simulink model "pTopModel"  (R2021a)
settings: Solver=FixedStepAuto  StartTime=0.0  StopTime=200  FixedStep=Ts  RelTol=1e-3
values from neighbouring files (symbols this model uses):
  C = 1 - 0.287*log(gamma)    [SIDWaveGenerator.m]
  Ef = rho*g^2*D*A^2/(4*w)    [SIDWaveGenerator.m]
  Ts = 1/1000    (= 0.001)    [FOSTWINctrlPost.m]    (also in initModels_GUI.m)
undefined symbols (not defined in the file or in its folder): Aft, AveragePower, Bow, dataID_twin, pcktID, SimStateMsg, Total
libraries: simulink x19, slrealtimeutilitieslib x11, slrealtimeethercatlib x6, slrealtimeiplib x3, slrealtimeloglib x2, dspstat3 x1
settings Model: SimulationMode=external  Creator=Johannes  LastModifiedBy=HWRL user
settings SolverCC: ConcurrentTasks=on  AlgebraicLoopSolver=TrustRegion  PositivePriorityOrder=on
settings DataIOCC: ExternalInput=Fexin.getElement(1),Fexin.getElement(2)  LoadExternalInput=on
settings OptimizationCC: BlockReduction=off  OptimizeBlockIOStorage=off
settings DebuggingCC: TasksWithSamePriorityMsg=none  SFMachineParentedDataDiag=warning
settings HardwareCC: ProdBitPerLong=64  ProdLongLongMode=on  ProdHWDeviceType=Intel->x86-64 (Linux 64)
settings RTWCC: Description=Simulink Real-Time  SystemTargetFile=slrealtime.tlc  TemplateMakefile=slrealtime_default_tmf  RTWVerbose=off  Toolchain=Simulink Real-Time Toolchain  BuildConfiguration=Faster Runs  CodeExecutionProfiling=on  TargetLang=C++

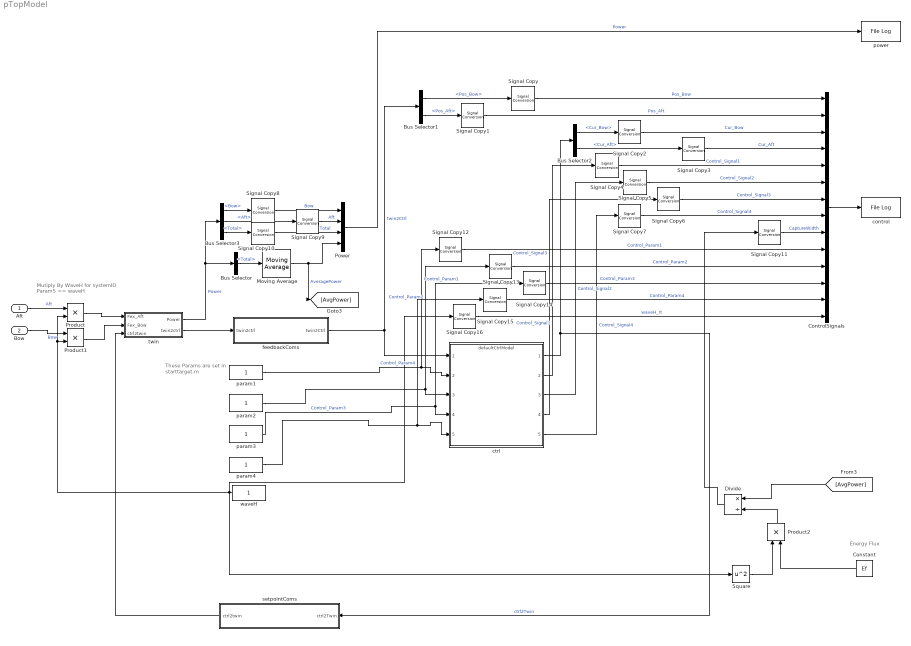
== system pTopModel ==
  note: Energy Flux
  note: Mutiply By WaveH for systemID
      | Param5 == waveH
  note: These Params are set in starttarget.m
  Aft : Inport  Interpolate=off
  Bow : Inport  Port=2  Interpolate=off
  Bus Selector : BusSelector  OutputSignals=Total
  Bus Selector1 : BusSelector  OutputSignals=Pos_Bow,Pos_Aft
  Bus Selector2 : BusSelector  OutputSignals=Cur_Bow,Cur_Aft
  Bus Selector3 : BusSelector  OutputSignals=Bow,Aft,Total
  Constant : Constant  Value=Ef  SampleTime=Ts
  ControlSignals : BusCreator  Inputs=14
  Divide : Product  Inputs=*/
  Moving Average : dspstat3/Moving Average  Method=Sliding window  ForgettingFactorPort=off  SpecifyWindowLength=on  WindowLength=numSteps  ForgettingFactor=0.9  SimulateUsing=Code generation
  Power : BusCreator  Inputs=Bow,Aft,Total,AveragePower
  Product : Product
  Product1 : Product
  Product2 : Product
  Signal Copy{,1..16} (17 alike) : SignalConversion  OverrideOpt=off
  Square : Math  Operator=square  SaturateOnIntegerOverflow=on
  control : slrealtimeloglib/File Log  decimation=10
      settings: SourceProductBaseCode=XP
  ctrl : ModelReference  ModelNameDialog=defaultCtrlModel  SimulationMode=Normal  ModelReferenceVersion=2.693
  feedbackComs : Subsystem  Variant=on  VariantControlMode=label  LabelModeActiveChoice=singleSpeedgoat
  param1 : Constant  OutDataTypeStr=Inherit: Inherit via back propagation  SampleTime=Ts
  param2 : Constant  SampleTime=Ts
  param3 : Constant  SampleTime=Ts
  param4 : Constant  VectorParams1D=off  SampleTime=Ts
  power : slrealtimeloglib/File Log  decimation=10
      settings: SourceProductBaseCode=XP
  setpointComs : Subsystem  Variant=on  VariantControlMode=label  LabelModeActiveChoice=singleSpeedgoat
  twin : Subsystem  Variant=on  VariantControlMode=label  LabelModeActiveChoice=systemID
  waveH : Constant  SampleTime=Ts
  wires:
  ctrl/1 -> Bus Selector2/1, setpointComs/1(ctrl2Twin)  "ctrl2Twin"
  feedbackComs/1(twin2Ctrl) -> ctrl/1, Bus Selector1/1  "twin2Ctrl"
  param1/1 -> ctrl/2, Signal Copy12/1  "Control_Param1"
  param2/1 -> ctrl/3, Signal Copy13/1  "Control_Param2"
  setpointComs/1(ctrl2twin) -> twin/3(ctrl2twin)
  twin/2(twin2ctrl) -> feedbackComs/1(twin2ctrl)
  param3/1 -> ctrl/4, Signal Copy14/1  "Control_Param3"
  ctrl/2 -> Signal Copy4/1  "Control_Signal1"
  ctrl/3 -> Signal Copy5/1  "Control_Signal2"
  ctrl/4 -> Signal Copy6/1  "Control_Signal3"
  ControlSignals/1 -> control/1
  param4/1 -> ctrl/5, Signal Copy15/1  "Control_Param4"
  Aft/1 -> Product/1  "Aft"
  Product/1 -> twin/1(Fex_Aft)
  Bow/1 -> Product1/1  "Bow"
  Product1/1 -> twin/2(Fex_Bow)
  ctrl/5 -> Signal Copy7/1  "Control_Signal4"
  twin/1(Power) -> Bus Selector3/1, Bus Selector/1  "Power"
  Bus Selector/1 -> Moving Average/1  "<Total>"
  Moving Average/1 -> [AvgPower], Power/4  "AveragePower"
  Power/1 -> power/1  "Power"
  Bus Selector1/1 -> Signal Copy/1  "<Pos_Bow>"
  Bus Selector1/2 -> Signal Copy1/1  "<Pos_Aft>"
  Bus Selector2/1 -> Signal Copy2/1  "<Cur_Bow>"
  Bus Selector2/2 -> Signal Copy3/1  "<Cur_Aft>"
  Bus Selector3/3 -> Signal Copy10/1  "<Total>"
  Bus Selector3/2 -> Signal Copy9/1  "<Aft>"
  Bus Selector3/1 -> Signal Copy8/1  "<Bow>"
  Signal Copy/1 -> ControlSignals/1  "Pos_Bow"
  Signal Copy1/1 -> ControlSignals/2  "Pos_Aft"
  Signal Copy2/1 -> ControlSignals/3  "Cur_Bow"
  Signal Copy3/1 -> ControlSignals/4  "Cur_Aft"
  Signal Copy4/1 -> ControlSignals/5  "Control_Signal1"
  Signal Copy5/1 -> ControlSignals/6  "Control_Signal2"
  Signal Copy6/1 -> ControlSignals/7  "Control_Signal3"
  Signal Copy7/1 -> ControlSignals/8  "Control_Signal4"
  Signal Copy8/1 -> Power/1  "Bow"
  Signal Copy9/1 -> Power/2  "Aft"
  Signal Copy10/1 -> Power/3  "Total"
  [AvgPower] -> Divide/1
  Constant/1 -> Product2/2
  Square/1 -> Product2/1
  Product2/1 -> Divide/2
  Divide/1 -> Signal Copy11/1
  Signal Copy11/1 -> ControlSignals/9  "CaptureWidth"
  Signal Copy12/1 -> ControlSignals/10  "Control_Param1"
  Signal Copy13/1 -> ControlSignals/11  "Control_Param2"
  Signal Copy14/1 -> ControlSignals/12  "Control_Param3"
  Signal Copy15/1 -> ControlSignals/13  "Control_Param4"
  Signal Copy16/1 -> ControlSignals/14  "waveH_rt"
  waveH/1 -> Square/1, Product/2, Product1/2, Signal Copy16/1

== system pTopModel/feedbackComs ==
  note: 1) Add Subsystem or Model blocks as valid variant choices.
      | 2) You cannot connect blocks at this level. At simulation, connectivity is automatically
      | determined, based on the active variant and port name matching.
  twin2ctrl : Inport
  nonRT : Subsystem  VariantControl=nonRT
  singleSpeedgoat : Subsystem  VariantControl=singleSpeedgoat
  twoSpeedgoats : Subsystem  VariantControl=twoSpeedgoats
  twin2Ctrl : Outport

== system pTopModel/setpointComs ==
  note: 1) Add Subsystem or Model blocks as valid variant choices.
      | 2) You cannot connect blocks at this level. At simulation, connectivity is automatically
      | determined, based on the active variant and port name matching.
  ctrl2Twin : Inport
  nonRT : Subsystem  VariantControl=nonRT
  singleSpeedgoat : Subsystem  VariantControl=singleSpeedgoat
  twoSpeedgoats : Subsystem  VariantControl=twoSpeedgoats
  ctrl2twin : Outport

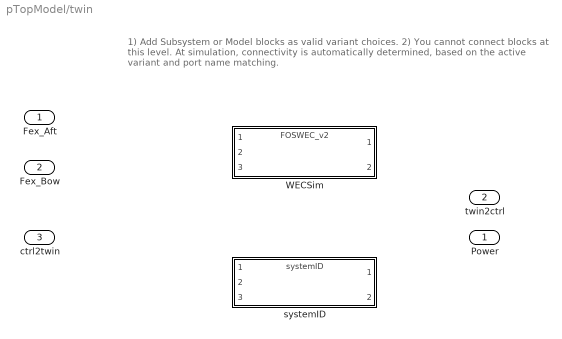
== system pTopModel/twin ==
  note: 1) Add Subsystem or Model blocks as valid variant choices.
      | 2) You cannot connect blocks at this level. At simulation, connectivity is automatically
      | determined, based on the active variant and port name matching.
  Fex_Aft : Inport
  Fex_Bow : Inport  Port=2
  ctrl2twin : Inport  Port=3
  WECSim : ModelReference  ModelNameDialog=FOSWEC_v2.slx  SimulationMode=Normal  VariantControl=WECSim  ModelReferenceVersion=3.577
  systemID : ModelReference  ModelNameDialog=systemID.slx  SimulationMode=Normal  VariantControl=systemID  ModelReferenceVersion=1.369
  Power : Outport
  twin2ctrl : Outport  Port=2

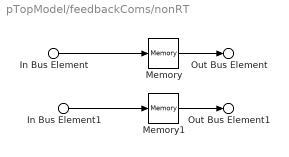
== system pTopModel/feedbackComs/nonRT ==
  In Bus Element : Inport  PortName=twin2ctrl  Element=Pos_Bow
  In Bus Element1 : Inport  PortName=twin2ctrl  Element=Pos_Aft
  Memory : Memory
  Memory1 : Memory
  Out Bus Element : Outport  PortName=twin2Ctrl  Element=Pos_Bow
  Out Bus Element1 : Outport  PortName=twin2Ctrl  Element=Pos_Aft
  wires:
  In Bus Element/1 -> Memory/1
  In Bus Element1/1 -> Memory1/1
  Memory1/1 -> Out Bus Element1/1
  Memory/1 -> Out Bus Element/1

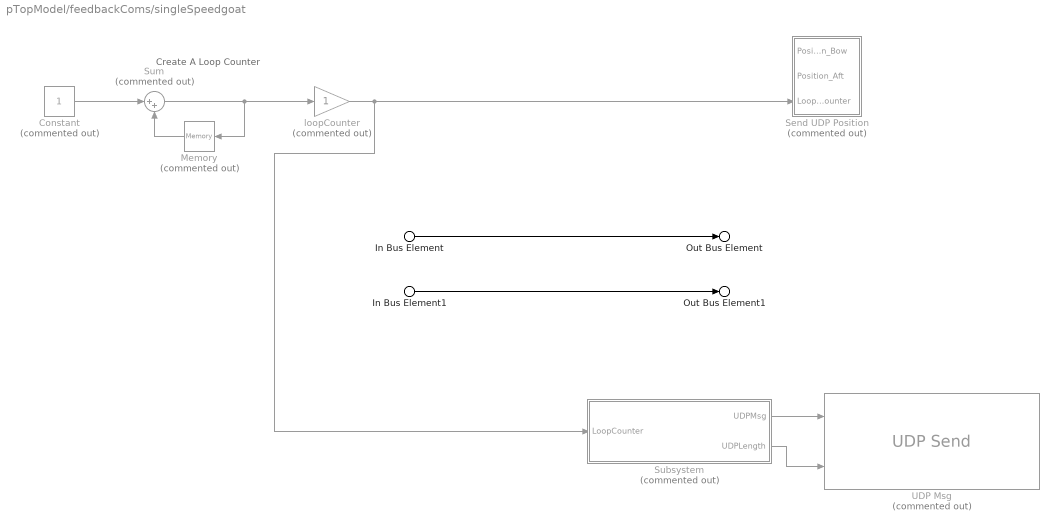
== system pTopModel/feedbackComs/singleSpeedgoat ==
  note: Create A Loop Counter
  In Bus Element : Inport  PortName=twin2ctrl  Element=Pos_Bow
  In Bus Element1 : Inport  PortName=twin2ctrl  Element=Pos_Aft
  Constant : Constant  Commented=on  SampleTime=Ts
  Memory : Memory  Commented=on
  Send UDP Position : Subsystem  Commented=on
  Subsystem : Subsystem  Commented=on
  Sum : Sum  Commented=on  Inputs=|++  OutDataTypeStr=uint32
  UDP Msg : slrealtimeiplib/UDP Send  Commented=on  useHostTargetConn=on  ipAddress=10.10.10.15  localPort=iotLocalMsgPort  toAddress=iotIPaddr  toPort=iotRemoteMsgPort  sampleTime=Ts
      settings: SourceProductBaseCode=XP
  loopCounter : Gain  Commented=on  ParamDataTypeStr=uint32  OutDataTypeStr=uint32
  Out Bus Element : Outport  PortName=twin2Ctrl  Element=Pos_Bow
  Out Bus Element1 : Outport  PortName=twin2Ctrl  Element=Pos_Aft
  wires:
  Subsystem/1(UDPMsg) -> UDP Msg/1
  Subsystem/2(UDPLength) -> UDP Msg/2
  In Bus Element/1 -> Out Bus Element/1
  In Bus Element1/1 -> Out Bus Element1/1
  Constant/1 -> Sum/1
  Sum/1 -> Memory/1, loopCounter/1
  Memory/1 -> Sum/2
  loopCounter/1 -> Subsystem/1(LoopCounter), Send UDP Position/3(LoopCounter)

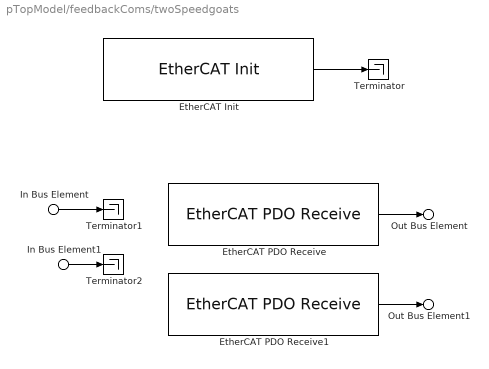
== system pTopModel/feedbackComs/twoSpeedgoats ==
  In Bus Element : Inport  PortName=twin2ctrl  Element=Pos_Bow
  In Bus Element1 : Inport  PortName=twin2ctrl  Element=Pos_Aft
  EtherCAT Init : slrealtimeethercatlib/EtherCAT Init  Priority=0  config_file=C:\Software\FOSTWIN\esi\FOSTWIN_Secondary1.xml  device_id=0  pci_bus=0  pci_slot=0  pci_function=0  portnum=1  initstate=2  dctuning=2  enaDebug=2  enaDC=on  errLink=off  masterDbg=off  stateChgDbg=off  baseClock=off  masterCfg=off  logFile='c:\dbglog.txt'  sample_time=0.001000  DCMode=0
      settings: SourceProductBaseCode=XP
  EtherCAT PDO Receive : slrealtimeethercatlib/EtherCAT PDO Receive  Priority=2  sig_name=Box 1 (EL6695-0002).IO Inputs.P2S01  sig_offset=328  sig_type=double  type_size=64  sig_dim=1  device_id=0  sample_time=0.001000
      settings: SourceProductBaseCode=XP
  EtherCAT PDO Receive1 : slrealtimeethercatlib/EtherCAT PDO Receive  Priority=2  sig_name=Box 1 (EL6695-0002).IO Inputs.P2S02  sig_offset=392  sig_type=double  type_size=64  sig_dim=1  device_id=0  sample_time=0.001000
      settings: SourceProductBaseCode=XP
  Terminator : Terminator
  Terminator1 : Terminator
  Terminator2 : Terminator
  Out Bus Element : Outport  PortName=twin2Ctrl  Element=Pos_Bow
  Out Bus Element1 : Outport  PortName=twin2Ctrl  Element=Pos_Aft
  wires:
  EtherCAT Init/1 -> Terminator/1
  EtherCAT PDO Receive/1 -> Out Bus Element/1
  In Bus Element/1 -> Terminator1/1
  EtherCAT PDO Receive1/1 -> Out Bus Element1/1
  In Bus Element1/1 -> Terminator2/1

== system pTopModel/setpointComs/nonRT ==
  In Bus Element : Inport  PortName=ctrl2Twin  Element=Cur_Bow
  In Bus Element1 : Inport  PortName=ctrl2Twin  Element=Cur_Aft
  Out Bus Element : Outport  PortName=ctrl2twin  Element=Cur_Bow
  Out Bus Element1 : Outport  PortName=ctrl2twin  Element=Cur_Aft
  wires:
  In Bus Element/1 -> Out Bus Element/1
  In Bus Element1/1 -> Out Bus Element1/1

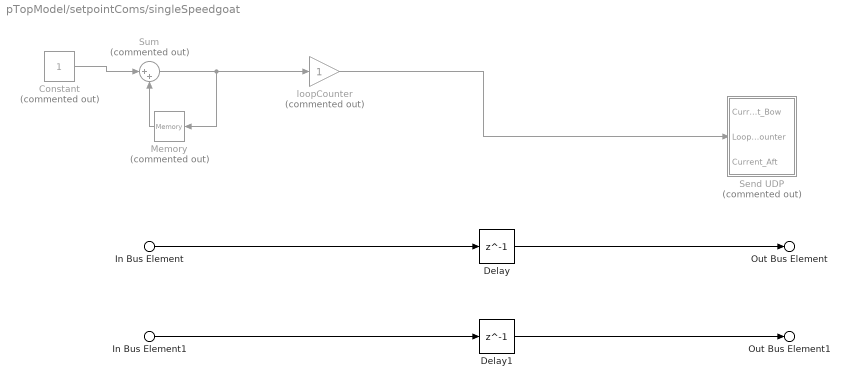
== system pTopModel/setpointComs/singleSpeedgoat ==
  In Bus Element : Inport  PortName=ctrl2Twin  Element=Cur_Bow
  In Bus Element1 : Inport  PortName=ctrl2Twin  Element=Cur_Aft
  Constant : Constant  Commented=on  SampleTime=Ts
  Delay : Delay  DelayLength=1
  Delay1 : Delay  DelayLength=1
  Memory : Memory  Commented=on
  Send UDP : Subsystem  Commented=on
  Sum : Sum  Commented=on  Inputs=|++  OutDataTypeStr=uint32
  loopCounter : Gain  Commented=on  ParamDataTypeStr=uint32  OutDataTypeStr=uint32
  Out Bus Element : Outport  PortName=ctrl2twin  Element=Cur_Bow
  Out Bus Element1 : Outport  PortName=ctrl2twin  Element=Cur_Aft
  wires:
  Constant/1 -> Sum/1
  In Bus Element/1 -> Delay/1
  In Bus Element1/1 -> Delay1/1
  Delay/1 -> Out Bus Element/1
  Delay1/1 -> Out Bus Element1/1
  Sum/1 -> Memory/1, loopCounter/1
  Memory/1 -> Sum/2
  loopCounter/1 -> Send UDP/2(LoopCounter)

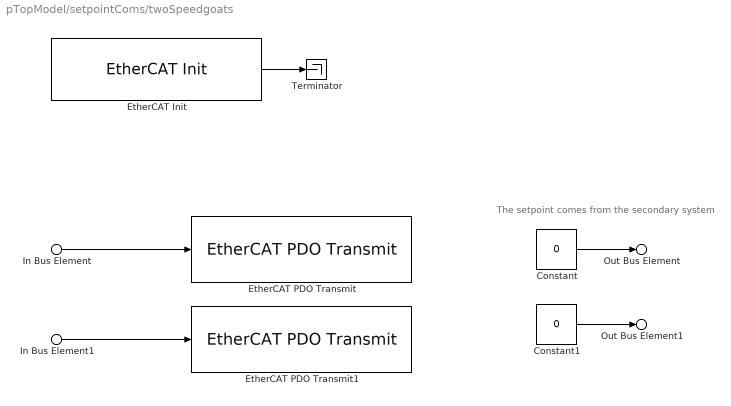
== system pTopModel/setpointComs/twoSpeedgoats ==
  note: The setpoint comes from the secondary system
  In Bus Element : Inport  PortName=ctrl2Twin  Element=Cur_Bow
  In Bus Element1 : Inport  PortName=ctrl2Twin  Element=Cur_Aft
  Constant : Constant  Value=0  VectorParams1D=off  SampleTime=-1
  Constant1 : Constant  Value=0  VectorParams1D=off  SampleTime=-1
  EtherCAT Init : slrealtimeethercatlib/EtherCAT Init  Priority=0  config_file=C:\Software\FOSTWIN\esi\FOSTWIN-Primary1.xml  device_id=0  pci_bus=0  pci_slot=0  pci_function=0  portnum=1  initstate=2  dctuning=0  enaDebug=0  enaDC=on  errLink=off  masterDbg=off  stateChgDbg=off  baseClock=off  masterCfg=off  logFile='c:\dbglog.txt'  sample_time=0.001000  DCMode=0
      settings: SourceProductBaseCode=XP
  EtherCAT PDO Transmit : slrealtimeethercatlib/EtherCAT PDO Transmit  Priority=3  sig_name=Term 2 (EL6695).IO Outputs.P2S01  sig_offset=312  sig_type=double  type_size=64  sig_dim=1  device_id=0  sample_time=0.001000
      settings: SourceProductBaseCode=XP
  EtherCAT PDO Transmit1 : slrealtimeethercatlib/EtherCAT PDO Transmit  Priority=3  sig_name=Term 2 (EL6695).IO Outputs.P2S02  sig_offset=376  sig_type=double  type_size=64  sig_dim=1  device_id=0  sample_time=0.001000
      settings: SourceProductBaseCode=XP
  Terminator : Terminator
  Out Bus Element : Outport  PortName=ctrl2twin  Element=Cur_Bow
  Out Bus Element1 : Outport  PortName=ctrl2twin  Element=Cur_Aft
  wires:
  Constant/1 -> Out Bus Element/1
  EtherCAT Init/1 -> Terminator/1
  Constant1/1 -> Out Bus Element1/1
  In Bus Element1/1 -> EtherCAT PDO Transmit1/1
  In Bus Element/1 -> EtherCAT PDO Transmit/1

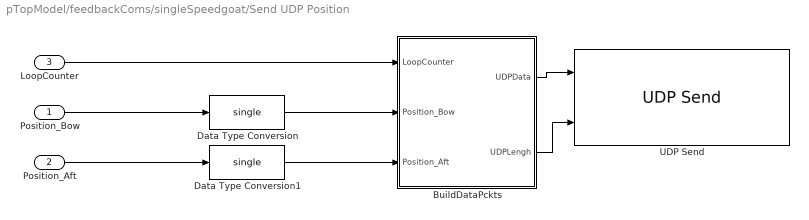
== system pTopModel/feedbackComs/singleSpeedgoat/Send UDP Position ==
  Position_Bow : Inport
  Position_Aft : Inport  Port=2
  LoopCounter : Inport  Port=3
  BuildDataPckts : Subsystem
  Data Type Conversion : DataTypeConversion  OutDataTypeStr=single
  Data Type Conversion1 : DataTypeConversion  OutDataTypeStr=single
  UDP Send : slrealtimeiplib/UDP Send  useHostTargetConn=on  ipAddress=10.10.10.15  localPort=iotLocalDataPort  toAddress=iotIPaddr  toPort=iotRemoteDataPort  sampleTime=Ts
      settings: SourceProductBaseCode=XP
  wires:
  BuildDataPckts/1(UDPData) -> UDP Send/1
  BuildDataPckts/2(UDPLengh) -> UDP Send/2
  Position_Bow/1 -> Data Type Conversion/1
  Data Type Conversion/1 -> BuildDataPckts/2(Position_Bow)
  Position_Aft/1 -> Data Type Conversion1/1
  Data Type Conversion1/1 -> BuildDataPckts/3(Position_Aft)
  LoopCounter/1 -> BuildDataPckts/1(LoopCounter)

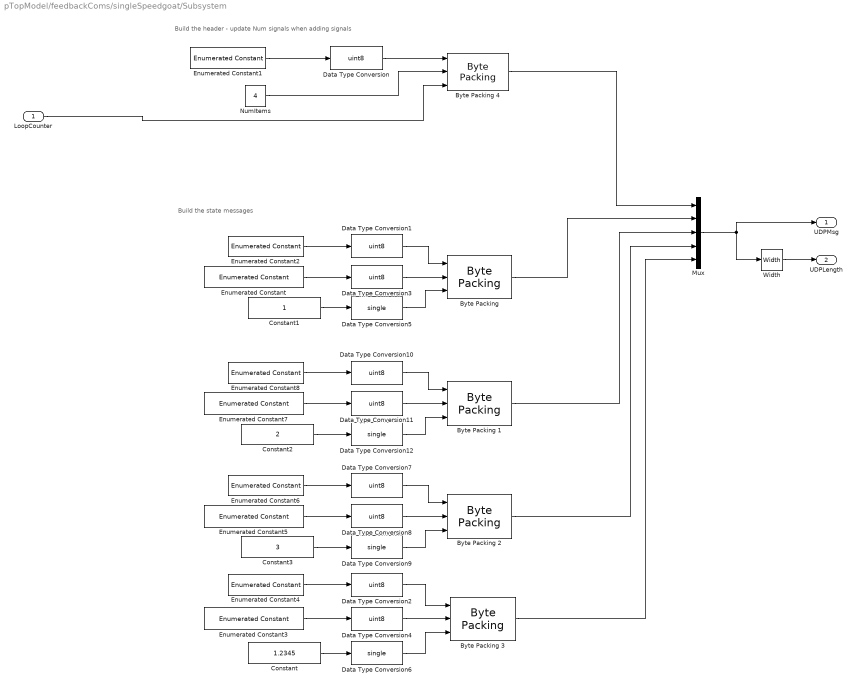
== system pTopModel/feedbackComs/singleSpeedgoat/Subsystem ==
  note: Build the state messages
  note: Build the header - update Num signals when adding signals
  LoopCounter : Inport
  Byte Packing {,1..4} (5 alike) : slrealtimeutilitieslib/Byte Packing
  Constant : Constant  Value=1.2345
  Constant1 : Constant
  Constant2 : Constant  Value=2
  Constant3 : Constant  Value=3
  Data Type Conversion{,1..4,7..8,10..11} (9 alike) : DataTypeConversion  OutDataTypeStr=uint8
  Data Type Conversion{5..6,9,12} (4 alike) : DataTypeConversion  OutDataTypeStr=single
  Enumerated Constant : simulink/Sources/Enumerated Constant  OutDataTypeStr=Enum: SimStateMsg  Value=SimStateMsg.eCATState  SampleTime=inf
  Enumerated Constant1 : simulink/Sources/Enumerated Constant  OutDataTypeStr=Enum: pcktID  Value=pcktID.header  SampleTime=inf
  Enumerated Constant{2,4,6,8} (4 alike) : simulink/Sources/Enumerated Constant  OutDataTypeStr=Enum: pcktID  Value=pcktID.stateMsg  SampleTime=inf
  Enumerated Constant3 : simulink/Sources/Enumerated Constant  OutDataTypeStr=Enum: SimStateMsg  Value=SimStateMsg.cpuTET  SampleTime=inf
  Enumerated Constant5 : simulink/Sources/Enumerated Constant  OutDataTypeStr=Enum: SimStateMsg  Value=SimStateMsg.eCATLastErr  SampleTime=inf
  Enumerated Constant7 : simulink/Sources/Enumerated Constant  OutDataTypeStr=Enum: SimStateMsg  Value=SimStateMsg.eCATErr  SampleTime=inf
  Mux : Mux  Inputs=5
  NumItems : Constant  Value=4  OutDataTypeStr=uint8
  Width : Width
  UDPMsg : Outport
  UDPLength : Outport  Port=2
  wires:
  Constant2/1 -> Data Type Conversion12/1
  NumItems/1 -> Byte Packing 4/2
  Data Type Conversion9/1 -> Byte Packing 2/3
  Constant3/1 -> Data Type Conversion9/1
  Enumerated Constant2/1 -> Data Type Conversion1/1
  Constant1/1 -> Data Type Conversion5/1
  Enumerated Constant7/1 -> Data Type Conversion11/1
  Data Type Conversion2/1 -> Byte Packing 3/1
  Enumerated Constant4/1 -> Data Type Conversion2/1
  Data Type Conversion4/1 -> Byte Packing 3/2
  Enumerated Constant6/1 -> Data Type Conversion7/1
  Mux/1 -> UDPMsg/1, Width/1
  Byte Packing 1/1 -> Mux/3
  Width/1 -> UDPLength/1
  Data Type Conversion5/1 -> "Byte Packing "/3
  Data Type Conversion12/1 -> Byte Packing 1/3
  "Byte Packing "/1 -> Mux/2
  Data Type Conversion3/1 -> "Byte Packing "/2
  Data Type Conversion6/1 -> Byte Packing 3/3
  Data Type Conversion8/1 -> Byte Packing 2/2
  Enumerated Constant3/1 -> Data Type Conversion4/1
  Enumerated Constant8/1 -> Data Type Conversion10/1
  Data Type Conversion11/1 -> Byte Packing 1/2
  Enumerated Constant5/1 -> Data Type Conversion8/1
  Data Type Conversion1/1 -> "Byte Packing "/1
  Byte Packing 4/1 -> Mux/1
  Byte Packing 3/1 -> Mux/5
  Byte Packing 2/1 -> Mux/4
  Enumerated Constant/1 -> Data Type Conversion3/1
  Constant/1 -> Data Type Conversion6/1
  Data Type Conversion10/1 -> Byte Packing 1/1
  Data Type Conversion/1 -> Byte Packing 4/1
  Data Type Conversion7/1 -> Byte Packing 2/1
  Enumerated Constant1/1 -> Data Type Conversion/1
  LoopCounter/1 -> Byte Packing 4/3

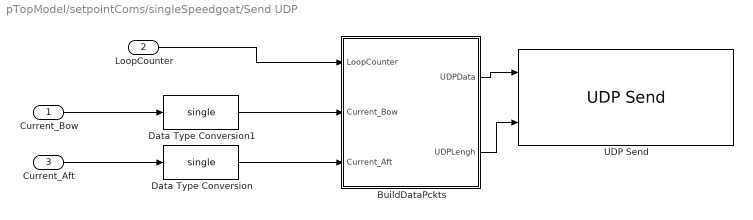
== system pTopModel/setpointComs/singleSpeedgoat/Send UDP ==
  Current_Bow : Inport
  LoopCounter : Inport  Port=2
  Current_Aft : Inport  Port=3
  BuildDataPckts : Subsystem
  Data Type Conversion : DataTypeConversion  OutDataTypeStr=single
  Data Type Conversion1 : DataTypeConversion  OutDataTypeStr=single
  UDP Send : slrealtimeiplib/UDP Send  useHostTargetConn=on  ipAddress=10.10.10.15  localPort=iotLocalDataPort  toAddress=iotIPaddr  toPort=iotRemoteDataPort  sampleTime=Ts
      settings: SourceProductBaseCode=XP
  wires:
  Current_Bow/1 -> Data Type Conversion1/1
  BuildDataPckts/1(UDPData) -> UDP Send/1
  BuildDataPckts/2(UDPLengh) -> UDP Send/2
  Current_Aft/1 -> Data Type Conversion/1
  LoopCounter/1 -> BuildDataPckts/1(LoopCounter)
  Data Type Conversion1/1 -> BuildDataPckts/2(Current_Bow)
  Data Type Conversion/1 -> BuildDataPckts/3(Current_Aft)

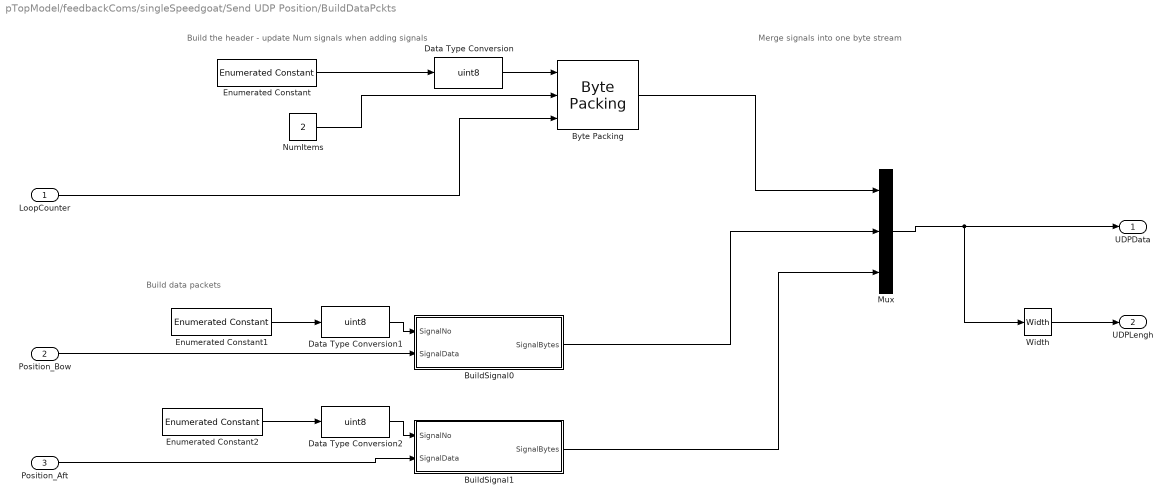
== system pTopModel/feedbackComs/singleSpeedgoat/Send UDP Position/BuildDataPckts ==
  note: Merge signals into one byte stream
  note: Build data packets
  note: Build the header - update Num signals when adding signals
  LoopCounter : Inport
  Position_Bow : Inport  Port=2  OutDataTypeStr=single
  Position_Aft : Inport  Port=3  OutDataTypeStr=single
  BuildSignal0 : Subsystem
  BuildSignal1 : Subsystem
  "Byte Packing " : slrealtimeutilitieslib/Byte Packing  MaskPackedDataType=uint8  MaskUnpackedDataTypes={'uint8','uint8','uint32'}  MaskAlignment=1
  Data Type Conversion : DataTypeConversion  OutDataTypeStr=uint8
  Data Type Conversion1 : DataTypeConversion  OutDataTypeStr=uint8
  Data Type Conversion2 : DataTypeConversion  OutDataTypeStr=uint8
  Enumerated Constant : simulink/Sources/Enumerated Constant  OutDataTypeStr=Enum: pcktID  Value=pcktID.header  SampleTime=inf
  Enumerated Constant1 : simulink/Sources/Enumerated Constant  OutDataTypeStr=Enum: dataID_twin  Value=dataID_twin.position_bow  SampleTime=inf
  Enumerated Constant2 : simulink/Sources/Enumerated Constant  OutDataTypeStr=Enum: dataID_twin  Value=dataID_twin.position_aft  SampleTime=inf
  Mux : Mux  Inputs=3
  NumItems : Constant  Value=2  OutDataTypeStr=uint8
  Width : Width
  UDPData : Outport
  UDPLengh : Outport  Port=2
  wires:
  Width/1 -> UDPLengh/1
  Position_Bow/1 -> BuildSignal0/2(SignalData)
  "Byte Packing "/1 -> Mux/1
  BuildSignal0/1(SignalBytes) -> Mux/2
  BuildSignal1/1(SignalBytes) -> Mux/3
  Mux/1 -> Width/1, UDPData/1
  Data Type Conversion/1 -> "Byte Packing "/1
  Enumerated Constant/1 -> Data Type Conversion/1
  NumItems/1 -> "Byte Packing "/2
  LoopCounter/1 -> "Byte Packing "/3
  Position_Aft/1 -> BuildSignal1/2(SignalData)
  Data Type Conversion1/1 -> BuildSignal0/1(SignalNo)
  Data Type Conversion2/1 -> BuildSignal1/1(SignalNo)
  Enumerated Constant1/1 -> Data Type Conversion1/1
  Enumerated Constant2/1 -> Data Type Conversion2/1

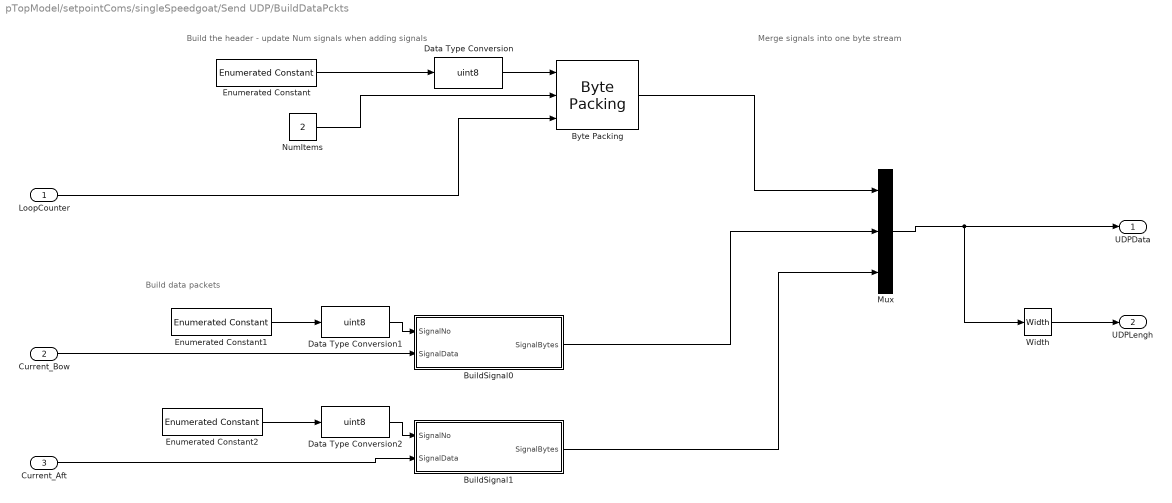
== system pTopModel/setpointComs/singleSpeedgoat/Send UDP/BuildDataPckts ==
  note: Merge signals into one byte stream
  note: Build data packets
  note: Build the header - update Num signals when adding signals
  LoopCounter : Inport
  Current_Bow : Inport  Port=2  OutDataTypeStr=single
  Current_Aft : Inport  Port=3  OutDataTypeStr=single
  BuildSignal0 : Subsystem
  BuildSignal1 : Subsystem
  "Byte Packing " : slrealtimeutilitieslib/Byte Packing  MaskPackedDataType=uint8  MaskUnpackedDataTypes={'uint8','uint8','uint32'}  MaskAlignment=1
  Data Type Conversion : DataTypeConversion  OutDataTypeStr=uint8
  Data Type Conversion1 : DataTypeConversion  OutDataTypeStr=uint8
  Data Type Conversion2 : DataTypeConversion  OutDataTypeStr=uint8
  Enumerated Constant : simulink/Sources/Enumerated Constant  OutDataTypeStr=Enum: pcktID  Value=pcktID.header  SampleTime=inf
  Enumerated Constant1 : simulink/Sources/Enumerated Constant  OutDataTypeStr=Enum: dataID_twin  Value=dataID_twin.current_bow  SampleTime=inf
  Enumerated Constant2 : simulink/Sources/Enumerated Constant  OutDataTypeStr=Enum: dataID_twin  Value=dataID_twin.current_aft  SampleTime=inf
  Mux : Mux  Inputs=3
  NumItems : Constant  Value=2  OutDataTypeStr=uint8
  Width : Width
  UDPData : Outport
  UDPLengh : Outport  Port=2
  wires:
  Width/1 -> UDPLengh/1
  Current_Bow/1 -> BuildSignal0/2(SignalData)
  "Byte Packing "/1 -> Mux/1
  BuildSignal0/1(SignalBytes) -> Mux/2
  BuildSignal1/1(SignalBytes) -> Mux/3
  Mux/1 -> Width/1, UDPData/1
  Data Type Conversion/1 -> "Byte Packing "/1
  Enumerated Constant/1 -> Data Type Conversion/1
  NumItems/1 -> "Byte Packing "/2
  LoopCounter/1 -> "Byte Packing "/3
  Current_Aft/1 -> BuildSignal1/2(SignalData)
  Data Type Conversion1/1 -> BuildSignal0/1(SignalNo)
  Data Type Conversion2/1 -> BuildSignal1/1(SignalNo)
  Enumerated Constant1/1 -> Data Type Conversion1/1
  Enumerated Constant2/1 -> Data Type Conversion2/1

== system pTopModel/feedbackComs/singleSpeedgoat/Send UDP Position/BuildDataPckts/BuildSignal0 ==
  SignalNo : Inport
  SignalData : Inport  Port=2
  "Byte Packing " : slrealtimeutilitieslib/Byte Packing  MaskPackedDataType=uint8  MaskUnpackedDataTypes={'uint8','uint8','single'}  MaskAlignment=1
  Data Type Conversion : DataTypeConversion  OutDataTypeStr=uint8
  Enumerated Constant : simulink/Sources/Enumerated Constant  OutDataTypeStr=Enum: pcktID  Value=pcktID.data  SampleTime=inf
  SignalBytes : Outport
  wires:
  SignalNo/1 -> "Byte Packing "/2
  SignalData/1 -> "Byte Packing "/3
  "Byte Packing "/1 -> SignalBytes/1
  Enumerated Constant/1 -> Data Type Conversion/1
  Data Type Conversion/1 -> "Byte Packing "/1

== system pTopModel/feedbackComs/singleSpeedgoat/Send UDP Position/BuildDataPckts/BuildSignal1 ==
  SignalNo : Inport
  SignalData : Inport  Port=2
  "Byte Packing " : slrealtimeutilitieslib/Byte Packing  MaskPackedDataType=uint8  MaskUnpackedDataTypes={'uint8','uint8','single'}  MaskAlignment=1
  Data Type Conversion : DataTypeConversion  OutDataTypeStr=uint8
  Enumerated Constant : simulink/Sources/Enumerated Constant  OutDataTypeStr=Enum: pcktID  Value=pcktID.data  SampleTime=inf
  SignalBytes : Outport
  wires:
  Data Type Conversion/1 -> "Byte Packing "/1
  Enumerated Constant/1 -> Data Type Conversion/1
  "Byte Packing "/1 -> SignalBytes/1
  SignalData/1 -> "Byte Packing "/3
  SignalNo/1 -> "Byte Packing "/2

== system pTopModel/setpointComs/singleSpeedgoat/Send UDP/BuildDataPckts/BuildSignal0 ==
  SignalNo : Inport
  SignalData : Inport  Port=2
  "Byte Packing " : slrealtimeutilitieslib/Byte Packing  MaskPackedDataType=uint8  MaskUnpackedDataTypes={'uint8','uint8','single'}  MaskAlignment=1
  Data Type Conversion : DataTypeConversion  OutDataTypeStr=uint8
  Enumerated Constant : simulink/Sources/Enumerated Constant  OutDataTypeStr=Enum: pcktID  Value=pcktID.data  SampleTime=inf
  SignalBytes : Outport
  wires:
  SignalNo/1 -> "Byte Packing "/2
  SignalData/1 -> "Byte Packing "/3
  "Byte Packing "/1 -> SignalBytes/1
  Enumerated Constant/1 -> Data Type Conversion/1
  Data Type Conversion/1 -> "Byte Packing "/1

== system pTopModel/setpointComs/singleSpeedgoat/Send UDP/BuildDataPckts/BuildSignal1 ==
  SignalNo : Inport
  SignalData : Inport  Port=2
  "Byte Packing " : slrealtimeutilitieslib/Byte Packing  MaskPackedDataType=uint8  MaskUnpackedDataTypes={'uint8','uint8','single'}  MaskAlignment=1
  Data Type Conversion : DataTypeConversion  OutDataTypeStr=uint8
  Enumerated Constant : simulink/Sources/Enumerated Constant  OutDataTypeStr=Enum: pcktID  Value=pcktID.data  SampleTime=inf
  SignalBytes : Outport
  wires:
  Data Type Conversion/1 -> "Byte Packing "/1
  Enumerated Constant/1 -> Data Type Conversion/1
  "Byte Packing "/1 -> SignalBytes/1
  SignalData/1 -> "Byte Packing "/3
  SignalNo/1 -> "Byte Packing "/2
